simulink model "twolink_robust"  (R2014a)
settings: Solver=ode45  StartTime=0.0  StopTime=5.0  RelTol=1e-3
settings Model: Creator=Serhat  LastModifiedBy=Serhat

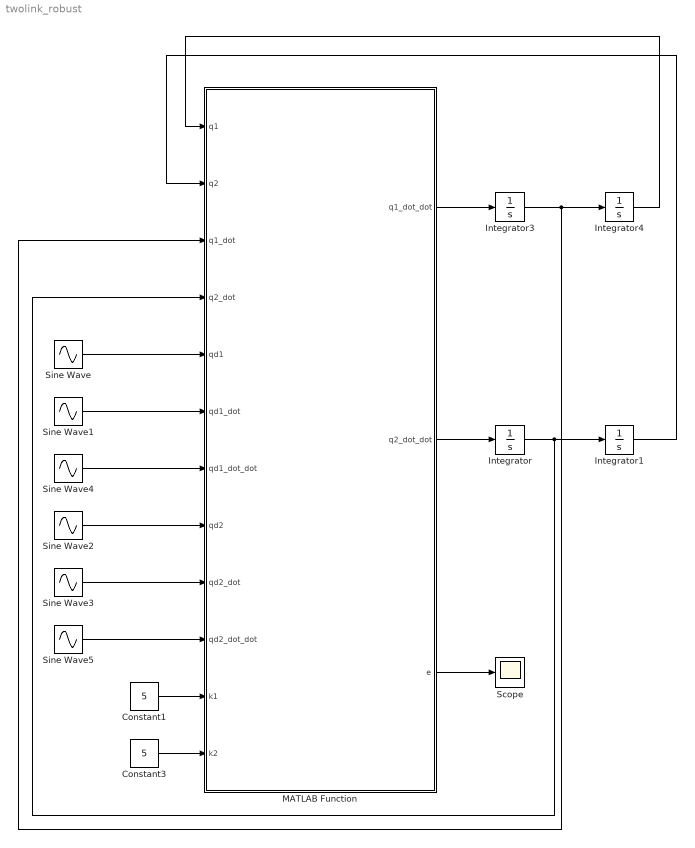
== system twolink_robust ==
  Constant1 : Constant  Value=5
  Constant3 : Constant  Value=5
  Integrator{,1,3..4} (4 alike) : Integrator  InitialCondition=10
  MATLAB Function : MATLAB Function  TreatAsAtomicUnit=on
  Scope : Scope
  Sine Wave : Sin  SampleTime=0
  Sine Wave1 : Sin  Phase=pi/2  SampleTime=0
  Sine Wave2 : Sin  SampleTime=0
  Sine Wave3 : Sin  Phase=pi/2  SampleTime=0
  Sine Wave4 : Sin  Phase=pi  SampleTime=0
  Sine Wave5 : Sin  Phase=pi  SampleTime=0
  wires:
  MATLAB Function/2(q2_dot_dot) -> Integrator/1
  Integrator/1 -> Integrator1/1, MATLAB Function/4(q2_dot)
  Integrator1/1 -> MATLAB Function/2(q2)
  MATLAB Function/1(q1_dot_dot) -> Integrator3/1
  Integrator3/1 -> Integrator4/1, MATLAB Function/3(q1_dot)
  Integrator4/1 -> MATLAB Function/1(q1)
  Sine Wave/1 -> MATLAB Function/5(qd1)
  Sine Wave1/1 -> MATLAB Function/6(qd1_dot)
  Sine Wave2/1 -> MATLAB Function/8(qd2)
  Sine Wave3/1 -> MATLAB Function/9(qd2_dot)
  MATLAB Function/3(e) -> Scope/1
  Sine Wave4/1 -> MATLAB Function/7(qd1_dot_dot)
  Sine Wave5/1 -> MATLAB Function/10(qd2_dot_dot)
  Constant1/1 -> MATLAB Function/11(k1)
  Constant3/1 -> MATLAB Function/12(k2)

== matlab function twolink_robust/MATLAB Function ==
  data: q1 input; q2 input; q1_dot input; q2_dot input; qd1 input; qd1_dot input; qd1_dot_dot input; qd2 input; qd2_dot input; qd2_dot_dot input; k1 input; k2 input; q1_dot_dot output; q2_dot_dot output; e output
function [q1_dot_dot, q2_dot_dot, e]= fcn(q1, q2, q1_dot, q2_dot,  qd1, qd1_dot, qd1_dot_dot, qd2, qd2_dot, qd2_dot_dot, k1, k2)
%#codegen

g = 9.8;

% Inertia Matrix
m1 = 1;
m2 = 1;

l1 = 0.40;
l2 = 0.40;

M12 = m2*l1*l2*cos(q2) + m2*(l2^2);
M21 = M12;
M22 = m2*(l2^2);
M11 = M22;

M = [ M11 M12 ; M21 M22];


% Centripedal Matrix
h = m2*l1*l2*sin(q2);

V11 = -h*q2_dot;
V12 = -h*q1_dot-h*q2_dot;
V21 = h*q1_dot;
V22 = 0;

V = [V11 V12; V21 V22 ];


% F
F1 = V(1)*q1_dot;
F2 = V(2)*q2_dot;

F = [ F1;  F2];


% Gravity
G1 = m1*l1*cos(q1) + m2*g*(l2*cos(q1+q2) + l1*cos(q1)); %???
G2 = m2*l2*g*cos(q1+q2);

G = [ G1; G2];


% Disturbance?
Td1 = k1*sign(q1_dot);
Td2 = k2 *sign(q2_dot);

Td = [ Td1; Td2];


% error & auxilary function

a = 3;
k = 15;

e11 = q1 - qd1;
e12 = q2 - qd2;

e = [e11; e12];

ed11 = q1_dot - qd1_dot;
ed12 = q2_dot - qd2_dot;

e_dot = [ed11; ed12];
r = e_dot + a*e;


q = [q1; q2];
q_dot = [q1_dot; q2_dot];
qd = [qd1; qd2];
qd_dot = [qd1_dot; qd2_dot];


T = -k*r;

q_dot_dot = (T - V*q_dot - G - transpose(F)*q_dot - Td) / 0.5;
q1_dot_dot = q_dot_dot(1);
q2_dot_dot = q_dot_dot(2);
